simulink model "Interface_algorithms"  (R2020b)
settings: Solver=ode1  StartTime=0.0  StopTime=1  RelTol=1e-3
libraries: powerlib x74
settings Model: Creator=Antero  LastModifiedBy=luans

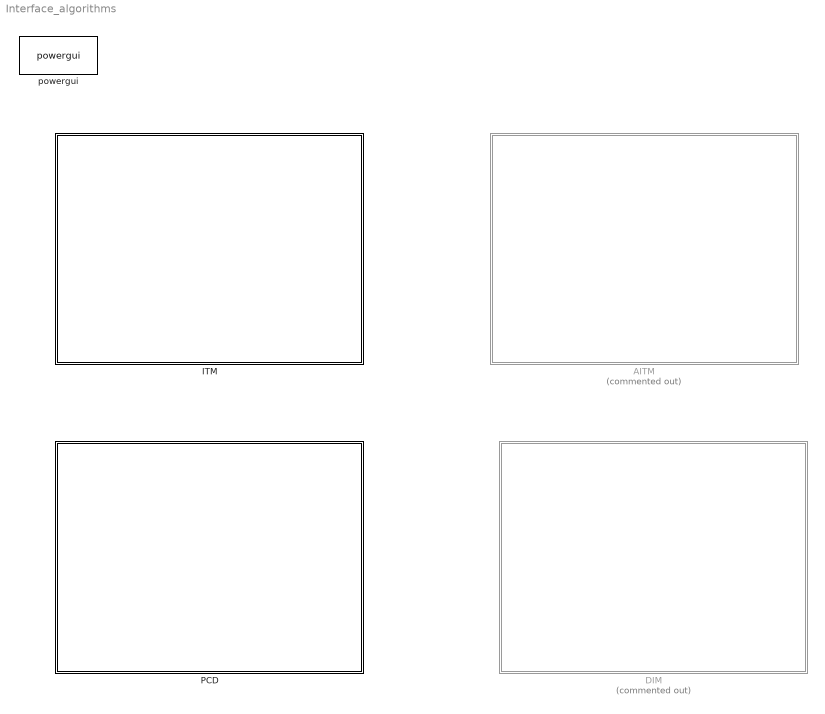
== system Interface_algorithms ==
  AITM : Subsystem  Commented=on
  DIM : Subsystem  Commented=on
  ITM : Subsystem
  PCD : Subsystem
  powergui : powerlib/powergui  Priority=1  SimulationMode=Discrete  SampleTime=50e-6  frequency=60  Iterations=50  frequencyindice=0  Pbase=100e6  ErrMax=1e-4  UnitsV=kV  UnitsW=MW  buscounter=0  FunctionMessages=off  echomessages=off  EnableUseOfTLC=off  CurrentSourceSwitches=off  DisableSnubberDevices=off  DisableRonSwitches=off  DisableVfSwitches=off  DisplayEquations=off  AutomaticDiscreteSolvers=off  SolverType=Tustin/Backward Euler (TBE)  Interpol=off  ExternalGateDelay=off  methode=off  Ts=100  x0status=blocks  SPID=on  SwTol=0  HookPort=off  NonlinearTolerance=1e-4  nMaxIteration=100  ContinueOnMaxIteration=off  RestoreLinks=warning  ResistiveCurrentMeasurement=off  Frange=[0:2:500]  Ylog=off  Xlog=on  ShowGrid=off  save=off  variable=ZData  structure=0  ZoomFFT=off  StartTime=0.0  cycles=1  DisplayStyle=1  fundamental=60  FreqAxis=off  MaxFrequency=1000  frequencyindicesteady=1  RmsSteady=1  display=off

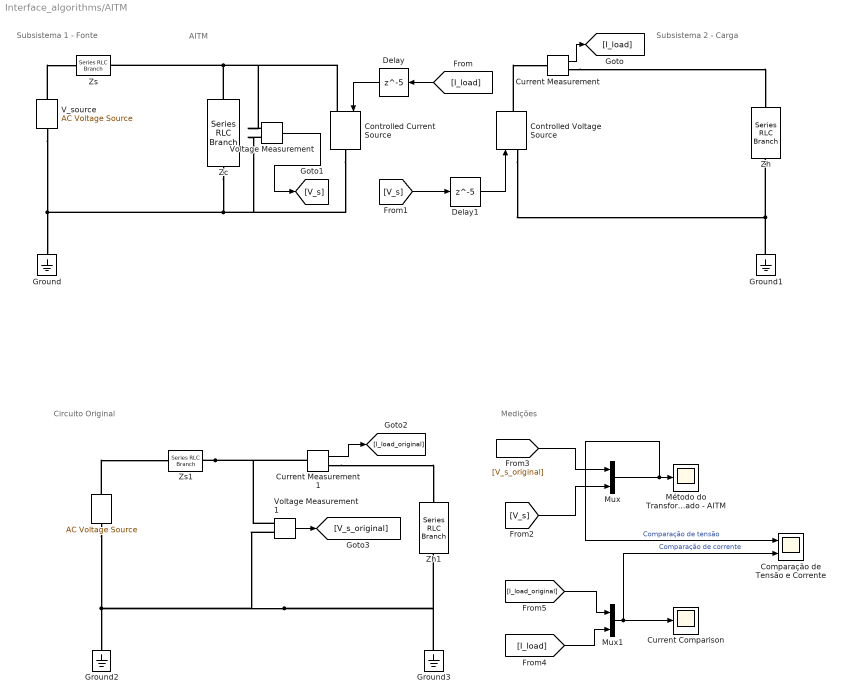
== system Interface_algorithms/AITM ==
  note: Subsistema 1 - Fonte
  note: Subsistema 2 - Carga
  note: Medições
  note: AITM
  note: Circuito Original
  " " : powerlib/Electrical Sources/AC Voltage Source  Amplitude=100  Phase=0  Frequency=60  SampleTime=0  Measurements=None  BusType=swing  Pref=10e3  Qref=0  Qmin=-inf  Qmax=+inf
  Comparação de Tensão e Corrente : Scope  NumInputPorts=2
  Controlled Current Source : powerlib/Electrical Sources/Controlled Current Source  Initialize=on  Source_Type=AC  Amplitude=0  Phase=0  Frequency=0  Measurements=None
  Controlled Voltage Source : powerlib/Electrical Sources/Controlled Voltage Source  Initialize=on  Source_Type=AC  Amplitude=0  Phase=0  Frequency=0  Measurements=None
  Current Comparison : Scope
  Current Measurement : powerlib/Measurements/Current Measurement  PhasorSimulation=off  OutputType=Complex  PSBequivalent=0
  Current Measurement1 : powerlib/Measurements/Current Measurement  PhasorSimulation=off  OutputType=Complex  PSBequivalent=0
  Delay : Delay  DelayLength=5
  Delay1 : Delay  DelayLength=5
  Ground{,1..3} (4 alike) : powerlib/Elements/Ground  LConnTagsString=a
  Mux : Mux  Inputs=2
  Mux1 : Mux  Inputs=2
  Método do Transformador Ideal Avançado - AITM : Scope
  V_source : powerlib/Electrical Sources/AC Voltage Source  Amplitude=100  Phase=0  Frequency=60  SampleTime=0  Measurements=None  BusType=swing  Pref=10e3  Qref=0  Qmin=-inf  Qmax=+inf
  Voltage Measurement : powerlib/Measurements/Voltage Measurement  PhasorSimulation=off  OutputType=Complex  PSBequivalent=0
  Voltage Measurement1 : powerlib/Measurements/Voltage Measurement  PhasorSimulation=off  OutputType=Complex  PSBequivalent=0
  Zc : powerlib/Elements/Series RLC Branch  LConnTagsString=__new0  RConnTagsString=__new0  BranchType=R  Resistance=20  Inductance=1e-3  SetiL0=off  InitialCurrent=0  Capacitance=1e-6  Setx0=off  InitialVoltage=0  Measurements=None
  Zh : powerlib/Elements/Series RLC Branch  LConnTagsString=__new0  RConnTagsString=__new0  BranchType=RL  Resistance=5  Inductance=1e-3  SetiL0=off  InitialCurrent=0  Capacitance=1e-6  Setx0=off  InitialVoltage=0  Measurements=None
  Zh1 : powerlib/Elements/Series RLC Branch  LConnTagsString=__new0  RConnTagsString=__new0  BranchType=RL  Resistance=5  Inductance=1e-3  SetiL0=off  InitialCurrent=0  Capacitance=1e-6  Setx0=off  InitialVoltage=0  Measurements=None
  Zs : powerlib/Elements/Series RLC Branch  LConnTagsString=__new0  RConnTagsString=__new0  BranchType=R  Resistance=2  Inductance=1e-3  SetiL0=off  InitialCurrent=0  Capacitance=1e-6  Setx0=off  InitialVoltage=0  Measurements=None
  Zs1 : powerlib/Elements/Series RLC Branch  LConnTagsString=__new0  RConnTagsString=__new0  BranchType=R  Resistance=2  Inductance=1e-3  SetiL0=off  InitialCurrent=0  Capacitance=1e-6  Setx0=off  InitialVoltage=0  Measurements=None
  wires:
  [I_load_original] -> Mux1/1
  Current Measurement/1 -> [I_load]
  [V_s] -> Delay1/1
  Delay/1 -> Controlled Current Source/1
  Voltage Measurement/1 -> [V_s]
  Voltage Measurement1/1 -> [V_s_original]
  [I_load] -> Delay/1
  Delay1/1 -> Controlled Voltage Source/1
  [V_s_original] -> Mux/1
  Mux/1 -> Comparação de Tensão e Corrente/1, Método do Transformador Ideal Avançado - AITM/1  "Comparação de tensão"
  [I_load] -> Mux1/2
  Mux1/1 -> Current Comparison/1, Comparação de Tensão e Corrente/2  "Comparação de corrente"
  Current Measurement1/1 -> [I_load_original]
  [V_s] -> Mux/2
  connections:
  " "/LConn1 -- Ground3/LConn1 -- Zh1/RConn1 -- Voltage Measurement1/LConn2 -- Ground2/LConn1
  Zs1/RConn1 -- Current Measurement1/LConn1 -- Voltage Measurement1/LConn1
  Controlled Current Source/LConn1 -- Voltage Measurement/LConn1 -- Zs/RConn1 -- Zc/LConn1
  Ground1/LConn1 -- Zh/RConn1 -- Controlled Voltage Source/LConn1
  V_source/LConn1 -- Zc/RConn1 -- Controlled Current Source/RConn1 -- Voltage Measurement/LConn2 -- Ground/LConn1
  V_source/RConn1 -- Zs/LConn1
  Controlled Voltage Source/RConn1 -- Current Measurement/LConn1
  Current Measurement/RConn1 -- Zh/LConn1
  Current Measurement1/RConn1 -- Zh1/LConn1
  " "/RConn1 -- Zs1/LConn1

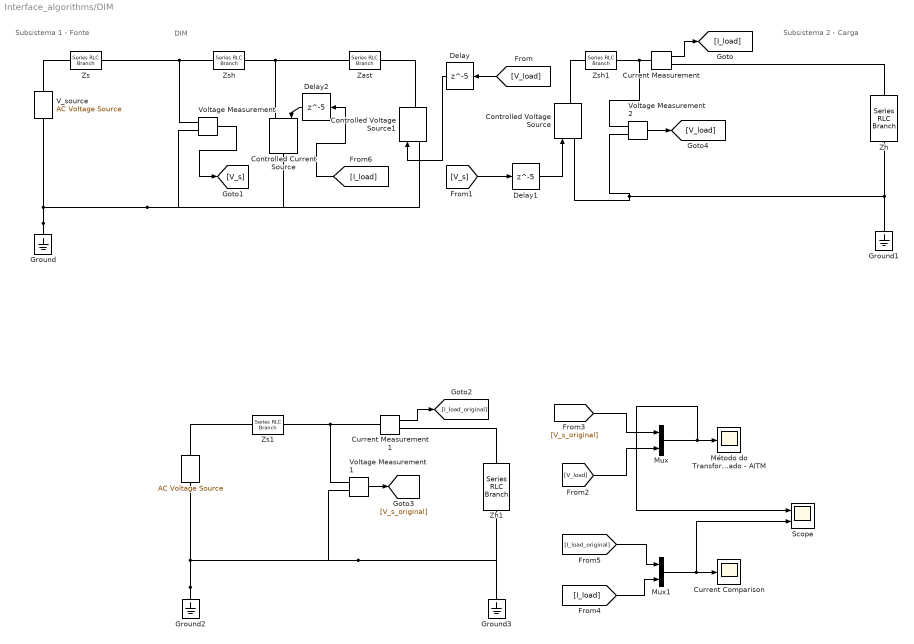
== system Interface_algorithms/DIM ==
  note: DIM
  note: Subsistema 2 - Carga
  note: Subsistema 1 - Fonte
  " " : powerlib/Electrical Sources/AC Voltage Source  Amplitude=100  Phase=0  Frequency=60  SampleTime=0  Measurements=None  BusType=swing  Pref=10e3  Qref=0  Qmin=-inf  Qmax=+inf
  Controlled Current Source : powerlib/Electrical Sources/Controlled Current Source  Initialize=on  Source_Type=AC  Amplitude=0  Phase=0  Frequency=0  Measurements=None
  Controlled Voltage Source : powerlib/Electrical Sources/Controlled Voltage Source  Initialize=on  Source_Type=AC  Amplitude=0  Phase=0  Frequency=0  Measurements=None
  Controlled Voltage Source1 : powerlib/Electrical Sources/Controlled Voltage Source  Initialize=on  Source_Type=AC  Amplitude=0  Phase=0  Frequency=0  Measurements=None
  Current Comparison : Scope
  Current Measurement : powerlib/Measurements/Current Measurement  PhasorSimulation=off  OutputType=Complex  PSBequivalent=0
  Current Measurement1 : powerlib/Measurements/Current Measurement  PhasorSimulation=off  OutputType=Complex  PSBequivalent=0
  Delay : Delay  DelayLength=5
  Delay1 : Delay  DelayLength=5
  Delay2 : Delay  DelayLength=5
  Ground{,1..3} (4 alike) : powerlib/Elements/Ground  LConnTagsString=a
  Mux : Mux  Inputs=2
  Mux1 : Mux  Inputs=2
  Método do Transformador Ideal Avançado - AITM : Scope
  Scope : Scope  NumInputPorts=2
  V_source : powerlib/Electrical Sources/AC Voltage Source  Amplitude=100  Phase=0  Frequency=60  SampleTime=0  Measurements=None  BusType=swing  Pref=10e3  Qref=0  Qmin=-inf  Qmax=+inf
  Voltage Measurement : powerlib/Measurements/Voltage Measurement  PhasorSimulation=off  OutputType=Complex  PSBequivalent=0
  Voltage Measurement1 : powerlib/Measurements/Voltage Measurement  PhasorSimulation=off  OutputType=Complex  PSBequivalent=0
  Voltage Measurement2 : powerlib/Measurements/Voltage Measurement  PhasorSimulation=off  OutputType=Complex  PSBequivalent=0
  Zast : powerlib/Elements/Series RLC Branch  LConnTagsString=__new0  RConnTagsString=__new0  BranchType=RL  Resistance=5  Inductance=1e-3  SetiL0=off  InitialCurrent=0  Capacitance=1e-6  Setx0=off  InitialVoltage=0  Measurements=None
  Zh : powerlib/Elements/Series RLC Branch  LConnTagsString=__new0  RConnTagsString=__new0  BranchType=RL  Resistance=5  Inductance=1e-3  SetiL0=off  InitialCurrent=0  Capacitance=1e-6  Setx0=off  InitialVoltage=0  Measurements=None
  Zh1 : powerlib/Elements/Series RLC Branch  LConnTagsString=__new0  RConnTagsString=__new0  BranchType=RL  Resistance=5  Inductance=1e-3  SetiL0=off  InitialCurrent=0  Capacitance=1e-6  Setx0=off  InitialVoltage=0  Measurements=None
  Zs : powerlib/Elements/Series RLC Branch  LConnTagsString=__new0  RConnTagsString=__new0  BranchType=R  Resistance=2  Inductance=1e-3  SetiL0=off  InitialCurrent=0  Capacitance=1e-6  Setx0=off  InitialVoltage=0  Measurements=None
  Zs1 : powerlib/Elements/Series RLC Branch  LConnTagsString=__new0  RConnTagsString=__new0  BranchType=R  Resistance=2  Inductance=1e-3  SetiL0=off  InitialCurrent=0  Capacitance=1e-6  Setx0=off  InitialVoltage=0  Measurements=None
  Zsh : powerlib/Elements/Series RLC Branch  LConnTagsString=__new0  RConnTagsString=__new0  BranchType=R  Resistance=1  Inductance=1e-3  SetiL0=off  InitialCurrent=0  Capacitance=1e-6  Setx0=off  InitialVoltage=0  Measurements=None
  Zsh1 : powerlib/Elements/Series RLC Branch  LConnTagsString=__new0  RConnTagsString=__new0  BranchType=R  Resistance=1  Inductance=1e-3  SetiL0=off  InitialCurrent=0  Capacitance=1e-6  Setx0=off  InitialVoltage=0  Measurements=None
  wires:
  Voltage Measurement/1 -> [V_s]
  [I_load] -> Mux1/2
  Current Measurement/1 -> [I_load]
  [I_load_original] -> Mux1/1
  Delay1/1 -> Controlled Voltage Source/1
  Voltage Measurement1/1 -> [V_s_original]
  [V_s_original] -> Mux/1
  [V_load] -> Mux/2
  Mux/1 -> Scope/1, Método do Transformador Ideal Avançado - AITM/1
  Mux1/1 -> Scope/2, Current Comparison/1
  [V_s] -> Delay1/1
  Current Measurement1/1 -> [I_load_original]
  [V_load] -> Delay/1
  Voltage Measurement2/1 -> [V_load]
  Delay/1 -> Controlled Voltage Source1/1
  Delay2/1 -> Controlled Current Source/1
  [I_load] -> Delay2/1
  connections:
  Ground2/LConn1 -- " "/LConn1 -- Voltage Measurement1/LConn2 -- Ground3/LConn1 -- Zh1/RConn1
  Ground/LConn1 -- Voltage Measurement/LConn2 -- Controlled Voltage Source1/LConn1 -- Controlled Current Source/RConn1 -- V_source/LConn1
  Voltage Measurement/LConn1 -- Zsh/LConn1 -- Zs/RConn1
  Controlled Voltage Source/LConn1 -- Voltage Measurement2/LConn2 -- Ground1/LConn1 -- Zh/RConn1
  Zsh1/RConn1 -- Voltage Measurement2/LConn1 -- Current Measurement/LConn1
  Voltage Measurement1/LConn1 -- Zs1/RConn1 -- Current Measurement1/LConn1
  V_source/RConn1 -- Zs/LConn1
  " "/RConn1 -- Zs1/LConn1
  Controlled Voltage Source/RConn1 -- Zsh1/LConn1
  Controlled Voltage Source1/RConn1 -- Zast/RConn1
  Current Measurement/RConn1 -- Zh/LConn1
  Current Measurement1/RConn1 -- Zh1/LConn1
  Zast/LConn1 -- Controlled Current Source/LConn1 -- Zsh/RConn1

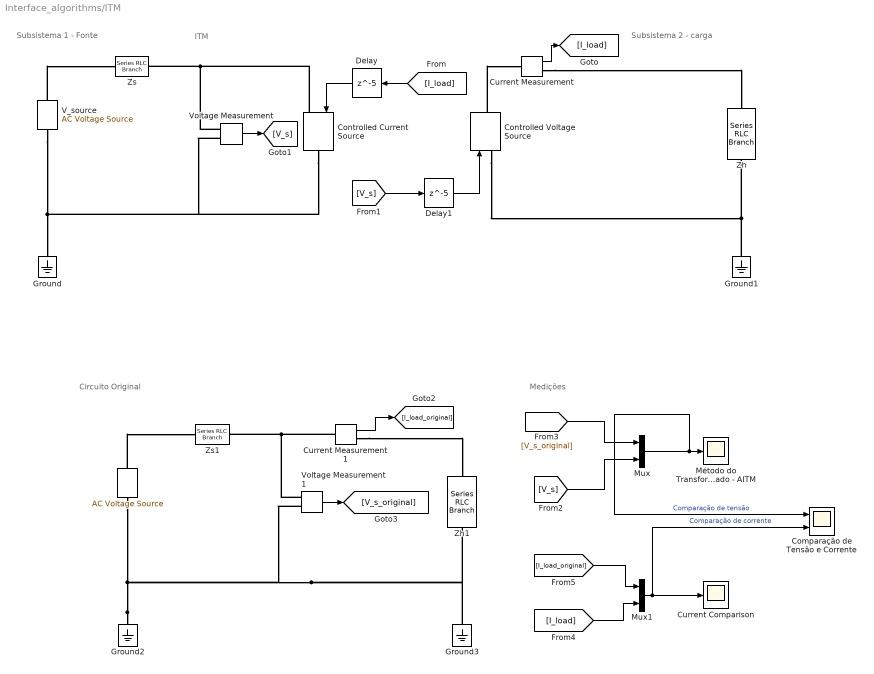
== system Interface_algorithms/ITM ==
  note: Subsistema 2 - carga
  note: ITM
  note: Subsistema 1 - Fonte
  note: Circuito Original
  note: Medições
  " " : powerlib/Electrical Sources/AC Voltage Source  Amplitude=100  Phase=0  Frequency=60  SampleTime=0  Measurements=None  BusType=swing  Pref=10e3  Qref=0  Qmin=-inf  Qmax=+inf
  Comparação de Tensão e Corrente : Scope  NumInputPorts=2
  Controlled Current Source : powerlib/Electrical Sources/Controlled Current Source  Initialize=on  Source_Type=AC  Amplitude=0  Phase=0  Frequency=0  Measurements=None
  Controlled Voltage Source : powerlib/Electrical Sources/Controlled Voltage Source  Initialize=on  Source_Type=AC  Amplitude=0  Phase=0  Frequency=0  Measurements=None
  Current Comparison : Scope
  Current Measurement : powerlib/Measurements/Current Measurement  PhasorSimulation=off  OutputType=Complex  PSBequivalent=0
  Current Measurement1 : powerlib/Measurements/Current Measurement  PhasorSimulation=off  OutputType=Complex  PSBequivalent=0
  Delay : Delay  DelayLength=5
  Delay1 : Delay  DelayLength=5
  Ground{,1..3} (4 alike) : powerlib/Elements/Ground  LConnTagsString=a
  Mux : Mux  Inputs=2
  Mux1 : Mux  Inputs=2
  Método do Transformador Ideal Avançado - AITM : Scope
  V_source : powerlib/Electrical Sources/AC Voltage Source  Amplitude=100  Phase=0  Frequency=60  SampleTime=0  Measurements=None  BusType=swing  Pref=10e3  Qref=0  Qmin=-inf  Qmax=+inf
  Voltage Measurement : powerlib/Measurements/Voltage Measurement  PhasorSimulation=off  OutputType=Complex  PSBequivalent=0
  Voltage Measurement1 : powerlib/Measurements/Voltage Measurement  PhasorSimulation=off  OutputType=Complex  PSBequivalent=0
  Zh : powerlib/Elements/Series RLC Branch  LConnTagsString=__new0  RConnTagsString=__new0  BranchType=RL  Resistance=5  Inductance=1e-3  SetiL0=off  InitialCurrent=0  Capacitance=1e-6  Setx0=off  InitialVoltage=0  Measurements=None
  Zh1 : powerlib/Elements/Series RLC Branch  LConnTagsString=__new0  RConnTagsString=__new0  BranchType=RL  Resistance=5  Inductance=1e-3  SetiL0=off  InitialCurrent=0  Capacitance=1e-6  Setx0=off  InitialVoltage=0  Measurements=None
  Zs : powerlib/Elements/Series RLC Branch  LConnTagsString=__new0  RConnTagsString=__new0  BranchType=R  Resistance=2  Inductance=1e-3  SetiL0=off  InitialCurrent=0  Capacitance=1e-6  Setx0=off  InitialVoltage=0  Measurements=None
  Zs1 : powerlib/Elements/Series RLC Branch  LConnTagsString=__new0  RConnTagsString=__new0  BranchType=R  Resistance=2  Inductance=1e-3  SetiL0=off  InitialCurrent=0  Capacitance=1e-6  Setx0=off  InitialVoltage=0  Measurements=None
  wires:
  Current Measurement/1 -> [I_load]
  [I_load] -> Delay/1
  Delay/1 -> Controlled Current Source/1
  Voltage Measurement/1 -> [V_s]
  [V_s] -> Delay1/1
  Delay1/1 -> Controlled Voltage Source/1
  Voltage Measurement1/1 -> [V_s_original]
  [I_load_original] -> Mux1/1
  [V_s_original] -> Mux/1
  Mux/1 -> Comparação de Tensão e Corrente/1, Método do Transformador Ideal Avançado - AITM/1  "Comparação de tensão"
  Current Measurement1/1 -> [I_load_original]
  [I_load] -> Mux1/2
  [V_s] -> Mux/2
  Mux1/1 -> Current Comparison/1, Comparação de Tensão e Corrente/2  "Comparação de corrente"
  connections:
  V_source/RConn1 -- Zs/LConn1
  V_source/LConn1 -- Controlled Current Source/RConn1 -- Voltage Measurement/LConn2 -- Ground/LConn1
  Controlled Current Source/LConn1 -- Voltage Measurement/LConn1 -- Zs/RConn1
  Ground1/LConn1 -- Zh/RConn1 -- Controlled Voltage Source/LConn1
  Controlled Voltage Source/RConn1 -- Current Measurement/LConn1
  Current Measurement/RConn1 -- Zh/LConn1
  Voltage Measurement1/LConn1 -- Zs1/RConn1 -- Current Measurement1/LConn1
  Ground2/LConn1 -- " "/LConn1 -- Ground3/LConn1 -- Zh1/RConn1 -- Voltage Measurement1/LConn2
  Current Measurement1/RConn1 -- Zh1/LConn1
  " "/RConn1 -- Zs1/LConn1

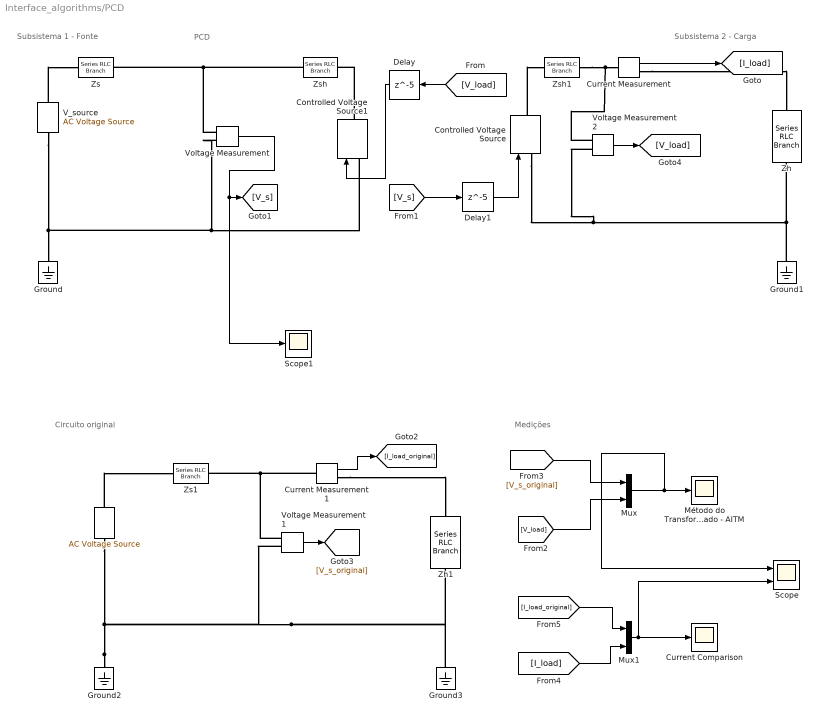
== system Interface_algorithms/PCD ==
  note: Subsistema 1 - Fonte
  note: Subsistema 2 - Carga
  note: Medições
  note: PCD
  note: Circuito original
  " " : powerlib/Electrical Sources/AC Voltage Source  Amplitude=100  Phase=0  Frequency=60  SampleTime=0  Measurements=None  BusType=swing  Pref=10e3  Qref=0  Qmin=-inf  Qmax=+inf
  Controlled Voltage Source : powerlib/Electrical Sources/Controlled Voltage Source  Initialize=on  Source_Type=AC  Amplitude=0  Phase=0  Frequency=0  Measurements=None
  Controlled Voltage Source1 : powerlib/Electrical Sources/Controlled Voltage Source  Initialize=on  Source_Type=AC  Amplitude=0  Phase=0  Frequency=0  Measurements=None
  Current Comparison : Scope
  Current Measurement : powerlib/Measurements/Current Measurement  PhasorSimulation=off  OutputType=Complex  PSBequivalent=0
  Current Measurement1 : powerlib/Measurements/Current Measurement  PhasorSimulation=off  OutputType=Complex  PSBequivalent=0
  Delay : Delay  DelayLength=5
  Delay1 : Delay  DelayLength=5
  Ground{,1..3} (4 alike) : powerlib/Elements/Ground  LConnTagsString=a
  Mux : Mux  Inputs=2
  Mux1 : Mux  Inputs=2
  Método do Transformador Ideal Avançado - AITM : Scope
  Scope : Scope  NumInputPorts=2
  Scope1 : Scope
  V_source : powerlib/Electrical Sources/AC Voltage Source  Amplitude=100  Phase=0  Frequency=60  SampleTime=0  Measurements=None  BusType=swing  Pref=10e3  Qref=0  Qmin=-inf  Qmax=+inf
  Voltage Measurement : powerlib/Measurements/Voltage Measurement  PhasorSimulation=off  OutputType=Complex  PSBequivalent=0
  Voltage Measurement1 : powerlib/Measurements/Voltage Measurement  PhasorSimulation=off  OutputType=Complex  PSBequivalent=0
  Voltage Measurement2 : powerlib/Measurements/Voltage Measurement  PhasorSimulation=off  OutputType=Complex  PSBequivalent=0
  Zh : powerlib/Elements/Series RLC Branch  LConnTagsString=__new0  RConnTagsString=__new0  BranchType=RL  Resistance=2  Inductance=1e-3  SetiL0=off  InitialCurrent=0  Capacitance=1e-6  Setx0=off  InitialVoltage=0  Measurements=None
  Zh1 : powerlib/Elements/Series RLC Branch  LConnTagsString=__new0  RConnTagsString=__new0  BranchType=RL  Resistance=2  Inductance=1e-3  SetiL0=off  InitialCurrent=0  Capacitance=1e-6  Setx0=off  InitialVoltage=0  Measurements=None
  Zs : powerlib/Elements/Series RLC Branch  LConnTagsString=__new0  RConnTagsString=__new0  BranchType=R  Resistance=5  Inductance=1e-3  SetiL0=off  InitialCurrent=0  Capacitance=1e-6  Setx0=off  InitialVoltage=0  Measurements=None
  Zs1 : powerlib/Elements/Series RLC Branch  LConnTagsString=__new0  RConnTagsString=__new0  BranchType=R  Resistance=5  Inductance=1e-3  SetiL0=off  InitialCurrent=0  Capacitance=1e-6  Setx0=off  InitialVoltage=0  Measurements=None
  Zsh : powerlib/Elements/Series RLC Branch  LConnTagsString=__new0  RConnTagsString=__new0  BranchType=R  Resistance=1  Inductance=1e-3  SetiL0=off  InitialCurrent=0  Capacitance=1e-6  Setx0=off  InitialVoltage=0  Measurements=None
  Zsh1 : powerlib/Elements/Series RLC Branch  LConnTagsString=__new0  RConnTagsString=__new0  BranchType=R  Resistance=1  Inductance=1e-3  SetiL0=off  InitialCurrent=0  Capacitance=1e-6  Setx0=off  InitialVoltage=0  Measurements=None
  wires:
  [V_load] -> Mux/2
  Current Measurement1/1 -> [I_load_original]
  [V_s] -> Delay1/1
  Voltage Measurement1/1 -> [V_s_original]
  [V_s_original] -> Mux/1
  Mux1/1 -> Scope/2, Current Comparison/1
  [I_load_original] -> Mux1/1
  [I_load] -> Mux1/2
  Delay1/1 -> Controlled Voltage Source/1
  Voltage Measurement/1 -> Scope1/1, [V_s]
  Current Measurement/1 -> [I_load]
  Delay/1 -> Controlled Voltage Source1/1
  Mux/1 -> Scope/1, Método do Transformador Ideal Avançado - AITM/1
  [V_load] -> Delay/1
  Voltage Measurement2/1 -> [V_load]
  connections:
  Voltage Measurement1/LConn1 -- Zs1/RConn1 -- Current Measurement1/LConn1
  Voltage Measurement/LConn1 -- Zsh/LConn1 -- Zs/RConn1
  Ground2/LConn1 -- " "/LConn1 -- Ground3/LConn1 -- Zh1/RConn1 -- Voltage Measurement1/LConn2
  Voltage Measurement/LConn2 -- V_source/LConn1 -- Ground/LConn1 -- Controlled Voltage Source1/LConn1
  Controlled Voltage Source/LConn1 -- Voltage Measurement2/LConn2 -- Ground1/LConn1 -- Zh/RConn1
  Zsh1/RConn1 -- Voltage Measurement2/LConn1 -- Current Measurement/LConn1
  Current Measurement/RConn1 -- Zh/LConn1
  V_source/RConn1 -- Zs/LConn1
  " "/RConn1 -- Zs1/LConn1
  Current Measurement1/RConn1 -- Zh1/LConn1
  Controlled Voltage Source1/RConn1 -- Zsh/RConn1
  Controlled Voltage Source/RConn1 -- Zsh1/LConn1
